simulink model "SE3031HW10_sim_Mazza"  (R2013a)
settings: Solver=ode45  StartTime=0.0  StopTime=10.0  RelTol=1e-3
settings Model: Creator=mazzas  LastModifiedBy=mazzas

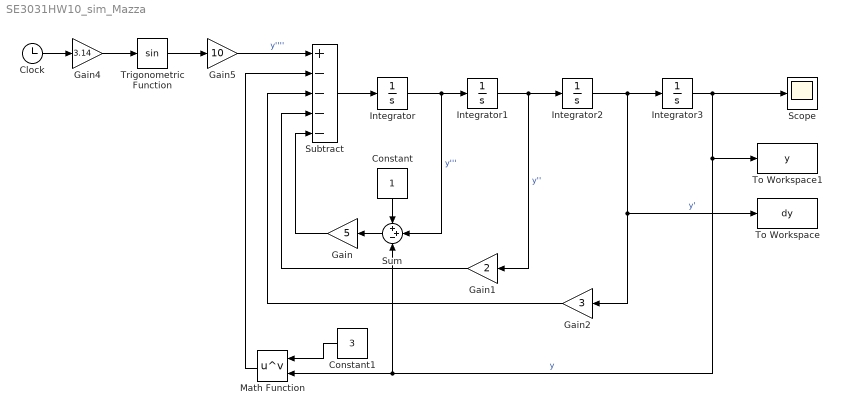
== system SE3031HW10_sim_Mazza ==
  Clock : Clock
  Constant : Constant
  Constant1 : Constant  Value=3
  Gain : Gain  Gain=5
  Gain1 : Gain  Gain=2
  Gain2 : Gain  Gain=3
  Gain4 : Gain  Gain=3.14
  Gain5 : Gain  Gain=10
  Integrator{,1..3} (4 alike) : Integrator
  Math Function : Math  Operator=pow  SaturateOnIntegerOverflow=on
  Scope : Scope
      settings: RequirementInfo="{}  %GIDa_3fe67d74_56cd_434f_8e8b_8bb64d505cfb"
  Subtract : Sum  Inputs=+----
  Sum : Sum  Inputs=++-
  To Workspace : ToWorkspace  VariableName=dy  SampleTime=-1
  To Workspace1 : ToWorkspace  VariableName=y  SampleTime=-1
  Trigonometric Function : Trigonometry
  wires:
  Integrator/1 -> Sum/2, Integrator1/1  "y'''"
  Integrator1/1 -> Gain1/1, Integrator2/1  "y''"
  Integrator2/1 -> To Workspace/1, Gain2/1, Integrator3/1  "y'"
  Integrator3/1 -> To Workspace1/1, Sum/3, Math Function/2, Scope/1  "y"
  Clock/1 -> Gain4/1
  Gain4/1 -> Trigonometric Function/1
  Trigonometric Function/1 -> Gain5/1
  Gain5/1 -> Subtract/1  "y''''"
  Gain1/1 -> Subtract/4
  Gain2/1 -> Subtract/3
  Subtract/1 -> Integrator/1
  Sum/1 -> Gain/1
  Constant/1 -> Sum/1
  Gain/1 -> Subtract/5
  Constant1/1 -> Math Function/1
  Math Function/1 -> Subtract/2
